simulink model "svpwm"  (R2022b)
settings: Solver=FixedStepAuto  StartTime=0.0  StopTime=10.0  FixedStep=1e-4  RelTol=1e-3
undefined symbols (not defined in the file): Pn
libraries: mcbplantlib x1, autolibpmsmexterior x1
settings Model: DataDictionary=svpwm.sldd  Creator=SSC  LastModifiedBy=SSC
settings OptimizationCC: DefaultParameterBehavior=Inlined  UseDivisionForNetSlopeComputation=on  GainParamInheritBuiltInType=on  UseFloatMulNetSlope=on  InlineInvariantSignals=on  PassReuseOutputArgsAs=Individual arguments  ZeroExternalMemoryAtStartup=off  ZeroInternalMemoryAtStartup=off  NoFixptDivByZeroProtection=on  EfficientFloat2IntCast=on  LifeSpan=1  OptimizeBlockOrder=speed  DifferentSizesBufferReuse=on  EfficientTunableParamExpr=on
settings DebuggingCC: ParameterTunabilityLossMsg=error
settings HardwareCC: ProdBitPerPointer=32  ProdBitPerSizeT=32  ProdBitPerPtrDiffT=32  ProdLargestAtomicInteger=Long  ProdLargestAtomicFloat=Double  ProdWordSize=32  ProdLongLongMode=on  ProdHWDeviceType=ARM Compatible->ARM Cortex-M
settings SFSimCC: MATLABDynamicMemAlloc=off
settings RTWCC: Description=Embedded Coder  SystemTargetFile=ert.tlc  TemplateMakefile=ert_default_tmf  GenerateReport=on  LaunchReport=on
settings CodeAppCC: ForceParamTrailComments=on  IgnoreCustomStorageClasses=off  OperatorAnnotations=on  SimulinkDataObjDesc=on  SFDataObjDesc=on  CustomSymbolStrGlobalVar=rt$N$M  CustomSymbolStrType=$N$M  CustomSymbolStrFcn=$N$M$F  CustomSymbolStrMacro=$N$M  InsertBlockDesc=on
settings ERTTargetCC: TargetLangStandard=C99 (ISO)  CodeReplacementLibrary=ARM Cortex-M  GenerateSampleERTMain=on  IncludeMdlTerminateFcn=off  CombineSignalStateStructs=on  SuppressErrorStatus=on  SupportAbsoluteTime=off  SupportNonFinite=off  SupportComplex=off  InlinedParameterPlacement=NonHierarchical  ERTCustomFileTemplate=example_file_process.tlc  ERTFilePackagingFormat=CompactWithDataFile

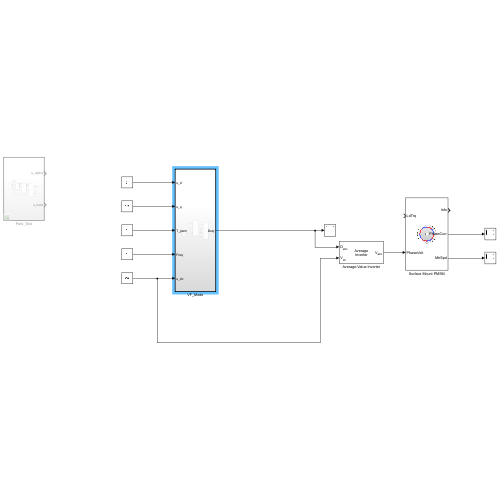
[thumbnail: Simulink's stored preview of the top-level diagram]
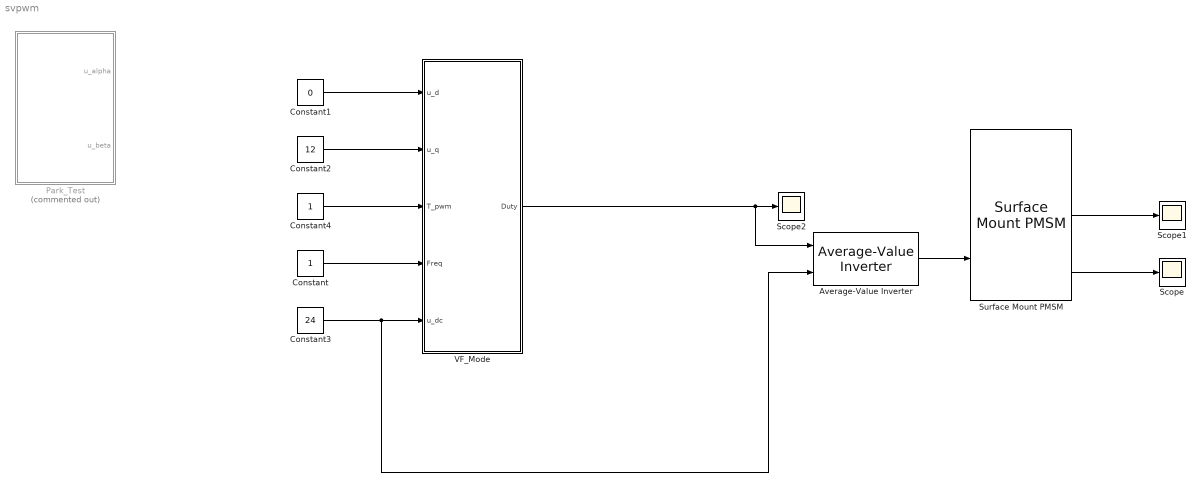
== system svpwm ==
  Average-Value Inverter : mcbplantlib/Average-Value Inverter
      settings: LibrarySourceBlock=mcblib/Electrical Systems/Inverters/Average-Value Inverter
  Constant : Constant
  Constant1 : Constant  Value=0
  Constant2 : Constant  Value=12
  Constant3 : Constant  Value=24
  Constant4 : Constant
  Park_Test : Subsystem  Commented=on  TreatAsAtomicUnit=on
  Scope : Scope
  Scope1 : Scope
  Scope2 : Scope
  Surface Mount PMSM : autolibpmsmexterior/Surface Mount PMSM  port_config=Torque  sim_type=Discrete  Ts=1e-4  P=Pn  Rs=Rs  Ldq_=L  KConstText=Permanent flux linkage constant (lambda_pm):  lambda_pm=flux  Ke=223  Kt=1.323  mechanical=[75e-6,8e-5,0]  idq0=[0 0]  theta_init=0  omega_init=0  KConst=flux  lambda_pm_calc=flux  RefBlkName='autolibpmsmexterior/Surface Mount PMSM'  aMode=5  Ldq="[0.0017      0.0017]"
  VF_Mode : Subsystem  TreatAsAtomicUnit=on
  wires:
  Constant3/1 -> Average-Value Inverter/2, VF_Mode/5(u_dc)
  Average-Value Inverter/1 -> Surface Mount PMSM/2
  Surface Mount PMSM/3 -> Scope/1
  Surface Mount PMSM/2 -> Scope1/1
  VF_Mode/1(Duty) -> Average-Value Inverter/1, Scope2/1
  Constant1/1 -> VF_Mode/1(u_d)
  Constant2/1 -> VF_Mode/2(u_q)
  Constant4/1 -> VF_Mode/3(T_pwm)
  Constant/1 -> VF_Mode/4(Freq)

== system svpwm/Park_Test ==
  AntiPark : Subsystem
  Clark : Subsystem
  Park : Subsystem
  Scope : Scope  NumInputPorts=3
  Scope1 : Scope  NumInputPorts=2
  Scope2 : Scope  NumInputPorts=2
  Scope3 : Scope  NumInputPorts=2
  ThreePhaseCurrGenerator : Subsystem
  u_alpha : Outport
  u_beta : Outport  Port=2
  wires:
  ThreePhaseCurrGenerator/1(ia) -> Scope/1, Clark/1(I_a)  "i_a"
  Clark/2(I_beta) -> Scope1/2, Park/2(i_beta)  "i_beta"
  Clark/1(I_alpha) -> Scope1/1, Park/1(i_alpha)  "i_alpha"
  ThreePhaseCurrGenerator/3(ic) -> Scope/3, Clark/3(I_c)  "i_c"
  ThreePhaseCurrGenerator/2(ib) -> Scope/2, Clark/2(I_b)  "i_b"
  ThreePhaseCurrGenerator/4(electric_theta) -> AntiPark/3(electric_theta), Park/3(electric_theta)  "electric_theta"
  Park/2(i_q) -> Scope3/2, AntiPark/2(u_q)  "i_q"
  Park/1(i_d) -> Scope3/1, AntiPark/1(u_d)  "i_d"
  AntiPark/1(u_alpha) -> u_alpha/1, Scope2/1
  AntiPark/2(u_beta) -> u_beta/1, Scope2/2

== system svpwm/VF_Mode ==
  u_d : Inport
  u_q : Inport  Port=2
  T_pwm : Inport  Port=3
  Freq : Inport  Port=4
  u_dc : Inport  Port=5
  AntiPark : Subsystem
  SVPWM : Subsystem
  ThreePhaseCurrGenerator : Subsystem
  Duty : Outport
  wires:
  u_dc/1 -> SVPWM/4(u_dc)
  ThreePhaseCurrGenerator/1(electric_theta) -> AntiPark/3(electric_theta)  "electric_theta"
  T_pwm/1 -> SVPWM/3(T_pwm)
  SVPWM/1(Duty) -> Duty/1
  u_q/1 -> AntiPark/2(u_q)
  AntiPark/2(u_beta) -> SVPWM/2(U_beta)
  Freq/1 -> ThreePhaseCurrGenerator/1(Freq)
  u_d/1 -> AntiPark/1(u_d)
  AntiPark/1(u_alpha) -> SVPWM/1(U_alpha)

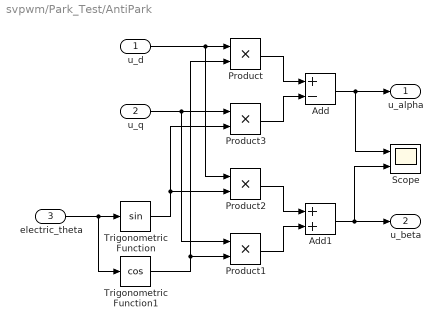
== system svpwm/Park_Test/AntiPark ==
  u_d : Inport
  u_q : Inport  Port=2
  electric_theta : Inport  Port=3
  Add : Sum  Inputs=+-
  Add1 : Sum
  Product{,1..3} (4 alike) : Product
  Scope : Scope  NumInputPorts=2
  Trigonometric Function : Trigonometry
  Trigonometric Function1 : Trigonometry  Operator=cos
  u_alpha : Outport
  u_beta : Outport  Port=2
  wires:
  electric_theta/1 -> Trigonometric Function1/1, Trigonometric Function/1
  u_d/1 -> Product2/1, Product/1
  Trigonometric Function1/1 -> Product/2, Product1/2
  u_q/1 -> Product1/1, Product3/1
  Trigonometric Function/1 -> Product2/2, Product3/2
  Product/1 -> Add/1
  Product3/1 -> Add/2
  Add/1 -> Scope/1, u_alpha/1
  Product2/1 -> Add1/1
  Product1/1 -> Add1/2
  Add1/1 -> Scope/2, u_beta/1

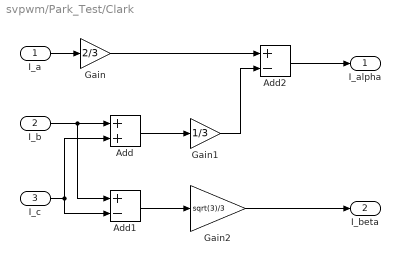
== system svpwm/Park_Test/Clark ==
  I_a : Inport
  I_b : Inport  Port=2
  I_c : Inport  Port=3
  Add : Sum
  Add1 : Sum  Inputs=+-
  Add2 : Sum  Inputs=+-
  Gain : Gain  Gain=2/3
  Gain1 : Gain  Gain=1/3
  Gain2 : Gain  Gain=sqrt(3)/3
  I_alpha : Outport
  I_beta : Outport  Port=2
  wires:
  I_a/1 -> Gain/1
  I_b/1 -> Add1/1, Add/1
  I_c/1 -> Add/2, Add1/2
  Add/1 -> Gain1/1
  Add1/1 -> Gain2/1
  Gain/1 -> Add2/1
  Gain1/1 -> Add2/2
  Add2/1 -> I_alpha/1
  Gain2/1 -> I_beta/1

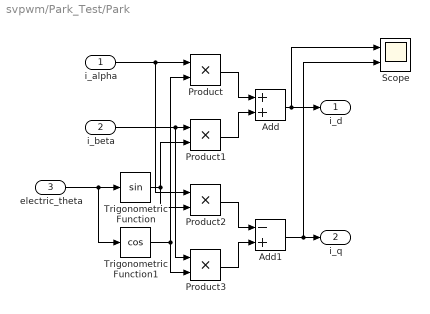
== system svpwm/Park_Test/Park ==
  i_alpha : Inport
  i_beta : Inport  Port=2
  electric_theta : Inport  Port=3
  Add : Sum
  Add1 : Sum  Inputs=-+
  Product{,1..3} (4 alike) : Product
  Scope : Scope  NumInputPorts=2
  Trigonometric Function : Trigonometry
  Trigonometric Function1 : Trigonometry  Operator=cos
  i_d : Outport
  i_q : Outport  Port=2
  wires:
  electric_theta/1 -> Trigonometric Function1/1, Trigonometric Function/1
  i_alpha/1 -> Product2/1, Product/1
  Trigonometric Function1/1 -> Product3/2, Product/2
  i_beta/1 -> Product3/1, Product1/1
  Trigonometric Function/1 -> Product2/2, Product1/2
  Product/1 -> Add/1
  Product1/1 -> Add/2
  Product2/1 -> Add1/1
  Product3/1 -> Add1/2
  Add/1 -> Scope/1, i_d/1
  Add1/1 -> Scope/2, i_q/1

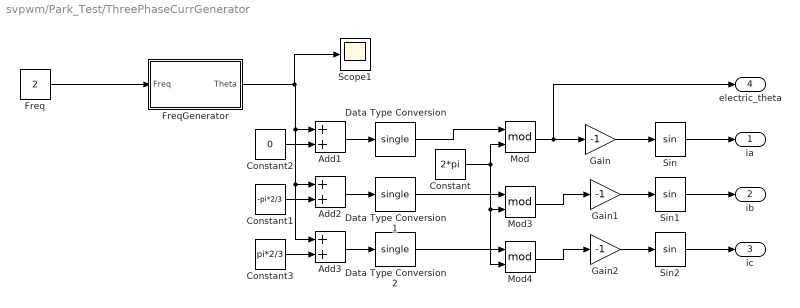
== system svpwm/Park_Test/ThreePhaseCurrGenerator ==
  Add1 : Sum  AccumDataTypeStr=single  OutDataTypeStr=single
  Add2 : Sum  AccumDataTypeStr=single  OutDataTypeStr=single
  Add3 : Sum  AccumDataTypeStr=single  OutDataTypeStr=single
  Constant : Constant  Value=2*pi  OutDataTypeStr=single
  Constant1 : Constant  Value=-pi*2/3  OutDataTypeStr=single
  Constant2 : Constant  Value=0  OutDataTypeStr=single
  Constant3 : Constant  Value=pi*2/3  OutDataTypeStr=single
  Data Type Conversion : DataTypeConversion  OutDataTypeStr=single  SaturateOnIntegerOverflow=off  RndMeth=Floor
  Data Type Conversion1 : DataTypeConversion  OutDataTypeStr=single  SaturateOnIntegerOverflow=off  RndMeth=Floor
  Data Type Conversion2 : DataTypeConversion  OutDataTypeStr=single  SaturateOnIntegerOverflow=off  RndMeth=Floor
  Freq : Constant  Value=2  OutDataTypeStr=single
  FreqGenerator : Subsystem
  Gain : Gain  Gain=-1
  Gain1 : Gain  Gain=-1
  Gain2 : Gain  Gain=-1
  Mod : Math  Operator=mod
  Mod3 : Math  Operator=mod
  Mod4 : Math  Operator=mod
  Scope1 : Scope
  Sin : Trigonometry  ApproximationMethod=Lookup
  Sin1 : Trigonometry  ApproximationMethod=Lookup
  Sin2 : Trigonometry  ApproximationMethod=Lookup
  ia : Outport
  ib : Outport  Port=2
  ic : Outport  Port=3
  electric_theta : Outport  Port=4
  wires:
  Sin2/1 -> ic/1
  Constant2/1 -> Add1/2
  Mod/1 -> electric_theta/1, Gain/1
  Constant/1 -> Mod4/2, Mod3/2, Mod/2
  Constant3/1 -> Add3/2
  Gain2/1 -> Sin2/1
  Constant1/1 -> Add2/2
  FreqGenerator/1(Theta) -> Scope1/1, Add3/1, Add2/1, Add1/1
  Sin/1 -> ia/1
  Sin1/1 -> ib/1
  Gain/1 -> Sin/1
  Add1/1 -> Data Type Conversion/1
  Data Type Conversion1/1 -> Mod3/1
  Mod3/1 -> Gain1/1
  Data Type Conversion/1 -> Mod/1
  Add2/1 -> Data Type Conversion1/1
  Add3/1 -> Data Type Conversion2/1
  Freq/1 -> FreqGenerator/1(Freq)
  Gain1/1 -> Sin1/1
  Data Type Conversion2/1 -> Mod4/1
  Mod4/1 -> Gain2/1

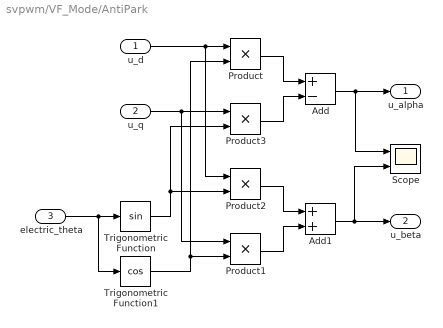
== system svpwm/VF_Mode/AntiPark ==
  u_d : Inport
  u_q : Inport  Port=2
  electric_theta : Inport  Port=3
  Add : Sum  Inputs=+-
  Add1 : Sum
  Product{,1..3} (4 alike) : Product
  Scope : Scope  NumInputPorts=2
  Trigonometric Function : Trigonometry
  Trigonometric Function1 : Trigonometry  Operator=cos
  u_alpha : Outport
  u_beta : Outport  Port=2
  wires:
  electric_theta/1 -> Trigonometric Function1/1, Trigonometric Function/1
  u_d/1 -> Product2/1, Product/1
  Trigonometric Function1/1 -> Product/2, Product1/2
  u_q/1 -> Product1/1, Product3/1
  Trigonometric Function/1 -> Product2/2, Product3/2
  Product/1 -> Add/1
  Product3/1 -> Add/2
  Add/1 -> Scope/1, u_alpha/1
  Product2/1 -> Add1/1
  Product1/1 -> Add1/2
  Add1/1 -> Scope/2, u_beta/1

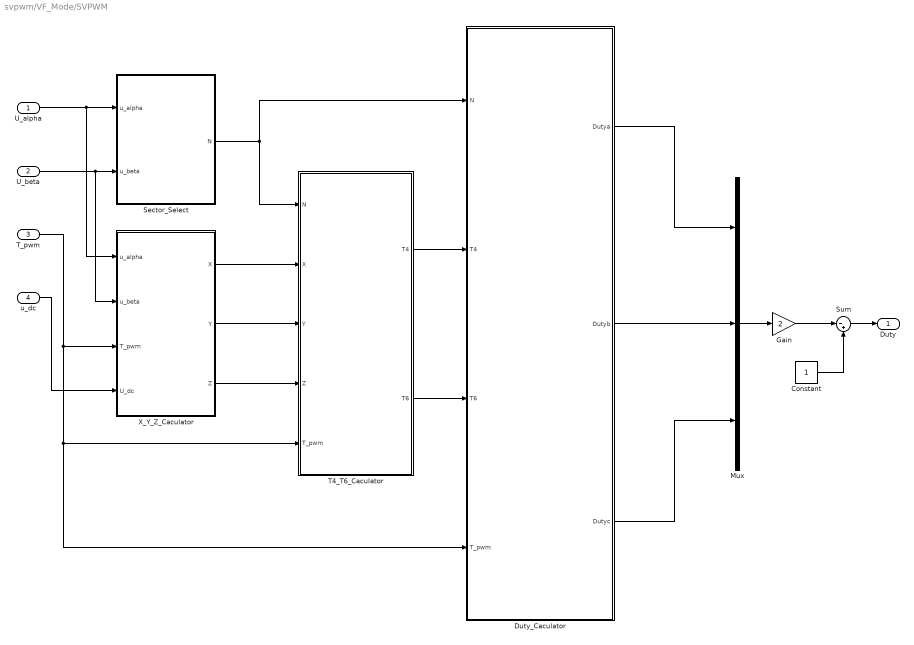
== system svpwm/VF_Mode/SVPWM ==
  U_alpha : Inport
  U_beta : Inport  Port=2
  T_pwm : Inport  Port=3
  u_dc : Inport  Port=4
  Constant : Constant
  Duty_Caculator : Subsystem
  Gain : Gain  Gain=2
  Mux : Mux  Inputs=3
  Sector_Select : Subsystem
  Sum : Sum  Inputs=|-+
  T4_T6_Caculator : Subsystem
  X_Y_Z_Caculator : Subsystem
  Duty : Outport
  wires:
  U_alpha/1 -> X_Y_Z_Caculator/1(u_alpha), Sector_Select/1(u_alpha)
  U_beta/1 -> X_Y_Z_Caculator/2(u_beta), Sector_Select/2(u_beta)
  T_pwm/1 -> Duty_Caculator/4(T_pwm), T4_T6_Caculator/5(T_pwm), X_Y_Z_Caculator/3(T_pwm)
  u_dc/1 -> X_Y_Z_Caculator/4(U_dc)
  X_Y_Z_Caculator/1(X) -> T4_T6_Caculator/2(X)
  X_Y_Z_Caculator/2(Y) -> T4_T6_Caculator/3(Y)
  X_Y_Z_Caculator/3(Z) -> T4_T6_Caculator/4(Z)
  Sector_Select/1(N) -> T4_T6_Caculator/1(N), Duty_Caculator/1(N)
  T4_T6_Caculator/2(T6) -> Duty_Caculator/3(T6)
  T4_T6_Caculator/1(T4) -> Duty_Caculator/2(T4)
  Duty_Caculator/2(Dutyb) -> Mux/2
  Duty_Caculator/1(Dutya) -> Mux/1
  Duty_Caculator/3(Dutyc) -> Mux/3
  Sum/1 -> Duty/1
  Constant/1 -> Sum/2
  Mux/1 -> Gain/1
  Gain/1 -> Sum/1

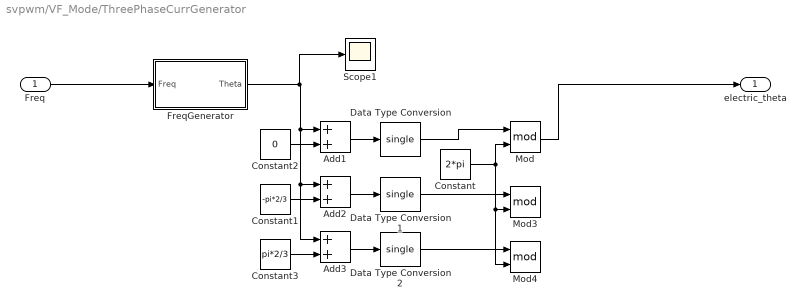
== system svpwm/VF_Mode/ThreePhaseCurrGenerator ==
  Freq : Inport
  Add1 : Sum  AccumDataTypeStr=single  OutDataTypeStr=single
  Add2 : Sum  AccumDataTypeStr=single  OutDataTypeStr=single
  Add3 : Sum  AccumDataTypeStr=single  OutDataTypeStr=single
  Constant : Constant  Value=2*pi  OutDataTypeStr=single
  Constant1 : Constant  Value=-pi*2/3  OutDataTypeStr=single
  Constant2 : Constant  Value=0  OutDataTypeStr=single
  Constant3 : Constant  Value=pi*2/3  OutDataTypeStr=single
  Data Type Conversion : DataTypeConversion  OutDataTypeStr=single  SaturateOnIntegerOverflow=off  RndMeth=Floor
  Data Type Conversion1 : DataTypeConversion  OutDataTypeStr=single  SaturateOnIntegerOverflow=off  RndMeth=Floor
  Data Type Conversion2 : DataTypeConversion  OutDataTypeStr=single  SaturateOnIntegerOverflow=off  RndMeth=Floor
  FreqGenerator : Subsystem
  Mod : Math  Operator=mod
  Mod3 : Math  Operator=mod
  Mod4 : Math  Operator=mod
  Scope1 : Scope
  electric_theta : Outport
  wires:
  Constant2/1 -> Add1/2
  Mod/1 -> electric_theta/1
  Constant/1 -> Mod4/2, Mod3/2, Mod/2
  Constant3/1 -> Add3/2
  Constant1/1 -> Add2/2
  FreqGenerator/1(Theta) -> Scope1/1, Add3/1, Add2/1, Add1/1
  Add1/1 -> Data Type Conversion/1
  Data Type Conversion1/1 -> Mod3/1
  Data Type Conversion/1 -> Mod/1
  Add2/1 -> Data Type Conversion1/1
  Add3/1 -> Data Type Conversion2/1
  Freq/1 -> FreqGenerator/1(Freq)
  Data Type Conversion2/1 -> Mod4/1

== system svpwm/Park_Test/ThreePhaseCurrGenerator/FreqGenerator ==
  Freq : Inport
  Gain : Gain  Gain=1/10e3*2*pi  OutDataTypeStr=single
  RangeLimit : Subsystem
  Sum : Sum  Inputs=|++  OutDataTypeStr=Inherit: Same as first input
  Unit Delay : UnitDelay  SampleTime=-1  HasFrameUpgradeWarning=on
  Theta : Outport
  wires:
  Freq/1 -> Gain/1
  RangeLimit/1(Theta) -> Theta/1, Unit Delay/1
  Gain/1 -> Sum/1
  Sum/1 -> RangeLimit/1(In)
  Unit Delay/1 -> Sum/2

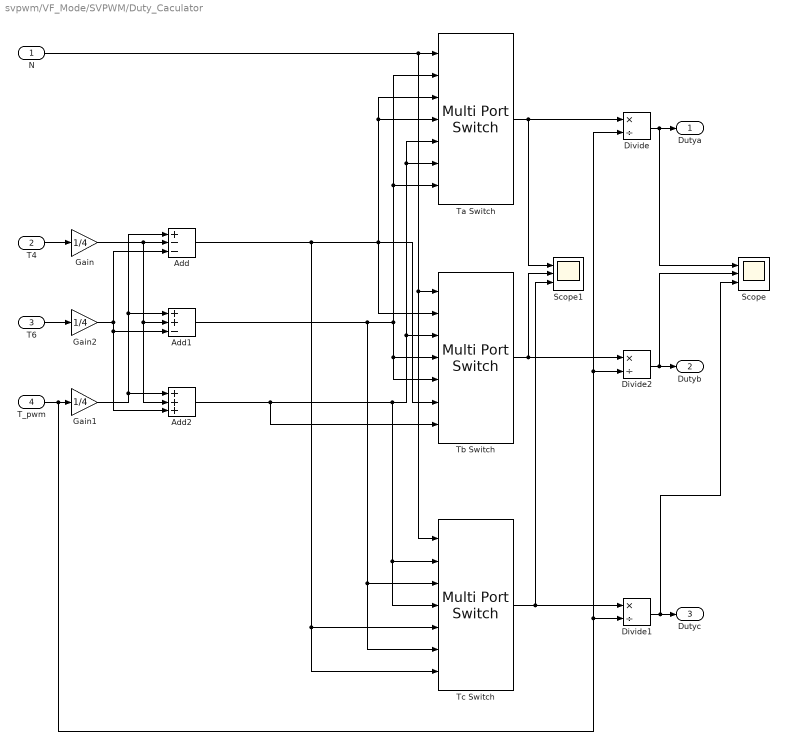
== system svpwm/VF_Mode/SVPWM/Duty_Caculator ==
  N : Inport
  T4 : Inport  Port=2
  T6 : Inport  Port=3
  T_pwm : Inport  Port=4
  Add : Sum  Inputs=+--
  Add1 : Sum  Inputs=++-
  Add2 : Sum  Inputs=+++
  Divide : Product  Inputs=*/
  Divide1 : Product  Inputs=*/
  Divide2 : Product  Inputs=*/
  Gain : Gain  Gain=1/4
  Gain1 : Gain  Gain=1/4
  Gain2 : Gain  Gain=1/4
  Scope : Scope  NumInputPorts=3
  Scope1 : Scope  NumInputPorts=3
  Ta Switch : MultiPortSwitch  Inputs=6  SaturateOnIntegerOverflow=off  InputSameDT=off
  Tb Switch : MultiPortSwitch  Inputs=6  SaturateOnIntegerOverflow=off  InputSameDT=off
  Tc Switch : MultiPortSwitch  Inputs=6  SaturateOnIntegerOverflow=off  InputSameDT=off
  Dutya : Outport
  Dutyb : Outport  Port=2
  Dutyc : Outport  Port=3
  wires:
  T4/1 -> Gain/1
  T6/1 -> Gain2/1
  T_pwm/1 -> Divide2/2, Divide/2, Divide1/2, Gain1/1
  Gain1/1 -> Add2/1, Add1/1, Add/1
  Gain/1 -> Add2/2, Add1/2, Add/2
  Gain2/1 -> Add2/3, Add1/3, Add/3
  N/1 -> Tc Switch/1, Tb Switch/1, Ta Switch/1
  Add/1 -> Tc Switch/7, Tc Switch/5, Tb Switch/6, Ta Switch/3, Ta Switch/4, Tb Switch/2
  Add1/1 -> Tc Switch/3, Tc Switch/6, Ta Switch/7, Ta Switch/2, Tb Switch/5, Tb Switch/4
  Add2/1 -> Tb Switch/7, Ta Switch/5, Ta Switch/6, Tb Switch/3, Tc Switch/4, Tc Switch/2
  Ta Switch/1 -> Scope1/1, Divide/1
  Tb Switch/1 -> Scope1/2, Divide2/1
  Tc Switch/1 -> Scope1/3, Divide1/1
  Divide/1 -> Scope/1, Dutya/1
  Divide1/1 -> Scope/3, Dutyc/1
  Divide2/1 -> Scope/2, Dutyb/1

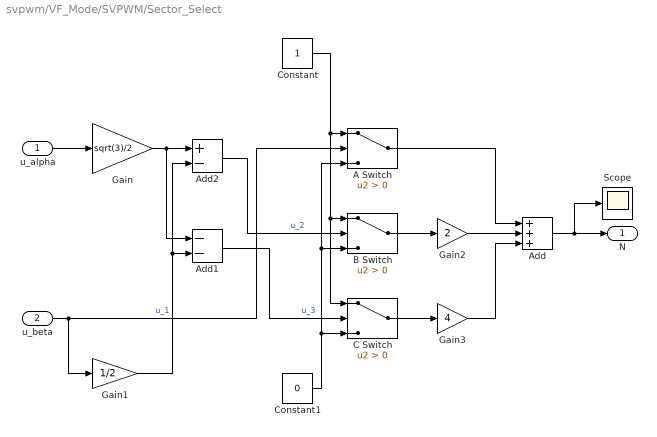
== system svpwm/VF_Mode/SVPWM/Sector_Select ==
  u_alpha : Inport
  u_beta : Inport  Port=2
  " A Switch" : Switch  Criteria=u2 > Threshold  SaturateOnIntegerOverflow=off  InputSameDT=off
  " B Switch" : Switch  Criteria=u2 > Threshold  SaturateOnIntegerOverflow=off  InputSameDT=off
  " C Switch" : Switch  Criteria=u2 > Threshold  SaturateOnIntegerOverflow=off  InputSameDT=off
  Add : Sum  Inputs=+++
  Add1 : Sum  Inputs=--
  Add2 : Sum  Inputs=+-
  Constant : Constant
  Constant1 : Constant  Value=0
  Gain : Gain  Gain=sqrt(3)/2
  Gain1 : Gain  Gain=1/2
  Gain2 : Gain  Gain=2
  Gain3 : Gain  Gain=4
  Scope : Scope
  N : Outport
  wires:
  Constant/1 -> " C Switch"/1, " B Switch"/1, " A Switch"/1
  Constant1/1 -> " C Switch"/3, " B Switch"/3, " A Switch"/3
  " A Switch"/1 -> Add/1
  Add/1 -> Scope/1, N/1
  " C Switch"/1 -> Gain3/1
  " B Switch"/1 -> Gain2/1
  u_beta/1 -> Gain1/1, " A Switch"/2  "u_1"
  u_alpha/1 -> Gain/1
  Gain/1 -> Add1/1, Add2/1
  Gain1/1 -> Add1/2, Add2/2
  Add2/1 -> " B Switch"/2  "u_2"
  Add1/1 -> " C Switch"/2  "u_3"
  Gain2/1 -> Add/2
  Gain3/1 -> Add/3

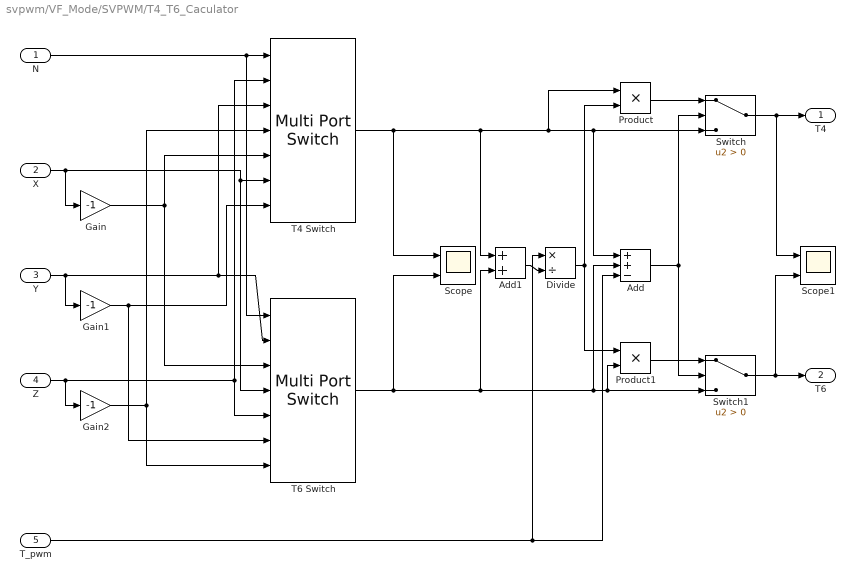
== system svpwm/VF_Mode/SVPWM/T4_T6_Caculator ==
  N : Inport
  X : Inport  Port=2
  Y : Inport  Port=3
  Z : Inport  Port=4
  T_pwm : Inport  Port=5
  Add : Sum  Inputs=++-
  Add1 : Sum
  Divide : Product  Inputs=*/
  Gain : Gain  Gain=-1
  Gain1 : Gain  Gain=-1
  Gain2 : Gain  Gain=-1
  Product : Product
  Product1 : Product
  Scope : Scope  NumInputPorts=2
  Scope1 : Scope  NumInputPorts=2
  Switch : Switch  Criteria=u2 > Threshold  SaturateOnIntegerOverflow=off  InputSameDT=off
  Switch1 : Switch  Criteria=u2 > Threshold  SaturateOnIntegerOverflow=off  InputSameDT=off
  T4 Switch : MultiPortSwitch  Inputs=6  SaturateOnIntegerOverflow=off  InputSameDT=off
  T6 Switch : MultiPortSwitch  Inputs=6  SaturateOnIntegerOverflow=off  InputSameDT=off
  T4 : Outport
  T6 : Outport  Port=2
  wires:
  Z/1 -> T4 Switch/2, T6 Switch/5, Gain2/1
  Y/1 -> Gain1/1, T4 Switch/3, T6 Switch/2
  X/1 -> T4 Switch/6, T6 Switch/4, Gain/1
  N/1 -> T6 Switch/1, T4 Switch/1
  Gain/1 -> T6 Switch/3, T4 Switch/5
  Gain2/1 -> T6 Switch/7, T4 Switch/4
  Gain1/1 -> T4 Switch/7, T6 Switch/6
  T4 Switch/1 -> Add1/1, Product/1, Add/1, Switch/3, Scope/1
  T6 Switch/1 -> Add1/2, Add/2, Switch1/3, Product1/2, Scope/2
  T_pwm/1 -> Add/3, Divide/1
  Add/1 -> Switch1/2, Switch/2
  Add1/1 -> Divide/2
  Product1/1 -> Switch1/1
  Product/1 -> Switch/1
  Divide/1 -> Product/2, Product1/1
  Switch/1 -> Scope1/1, T4/1
  Switch1/1 -> Scope1/2, T6/1

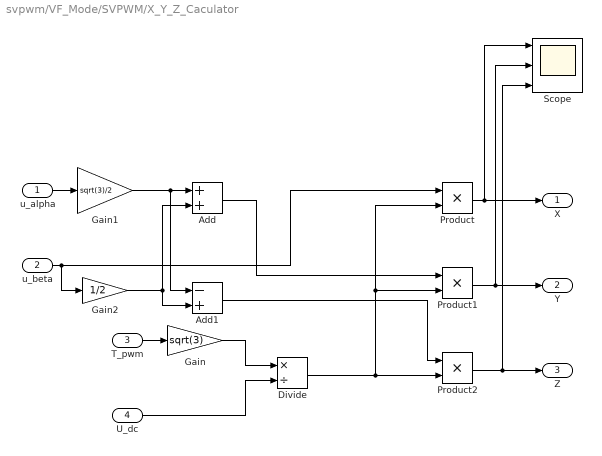
== system svpwm/VF_Mode/SVPWM/X_Y_Z_Caculator ==
  u_alpha : Inport
  u_beta : Inport  Port=2
  T_pwm : Inport  Port=3
  U_dc : Inport  Port=4
  Add : Sum
  Add1 : Sum  Inputs=-+
  Divide : Product  Inputs=*/
  Gain : Gain  Gain=sqrt(3)
  Gain1 : Gain  Gain=sqrt(3)/2
  Gain2 : Gain  Gain=1/2
  Product : Product
  Product1 : Product
  Product2 : Product
  Scope : Scope  NumInputPorts=3
  X : Outport
  Y : Outport  Port=2
  Z : Outport  Port=3
  wires:
  T_pwm/1 -> Gain/1
  U_dc/1 -> Divide/2
  Gain/1 -> Divide/1
  u_beta/1 -> Gain2/1, Product/1
  Divide/1 -> Product2/2, Product1/2, Product/2
  Product/1 -> Scope/1, X/1
  u_alpha/1 -> Gain1/1
  Gain1/1 -> Add1/1, Add/1
  Gain2/1 -> Add1/2, Add/2
  Add/1 -> Product1/1
  Product1/1 -> Scope/2, Y/1
  Add1/1 -> Product2/1
  Product2/1 -> Scope/3, Z/1

== system svpwm/VF_Mode/ThreePhaseCurrGenerator/FreqGenerator ==
  Freq : Inport
  Gain : Gain  Gain=1/10e3*2*pi  OutDataTypeStr=single
  RangeLimit : Subsystem
  Sum : Sum  Inputs=|++  OutDataTypeStr=Inherit: Same as first input
  Unit Delay : UnitDelay  SampleTime=-1  HasFrameUpgradeWarning=on
  Theta : Outport
  wires:
  Freq/1 -> Gain/1
  RangeLimit/1(Theta) -> Theta/1, Unit Delay/1
  Gain/1 -> Sum/1
  Sum/1 -> RangeLimit/1(In)
  Unit Delay/1 -> Sum/2

== system svpwm/Park_Test/ThreePhaseCurrGenerator/FreqGenerator/RangeLimit ==
  In : Inport
  Constant : Constant  Value=2*pi  OutDataTypeStr=single  SampleTime=-1
  Constant1 : Constant  Value=0  OutDataTypeStr=single  SampleTime=-1
  If : If  NumInputs=2  IfExpression=u1  ElseIfExpressions=u2
  If Action Subsystem1 : Subsystem  TreatAsAtomicUnit=on
  If Action Subsystem2 : Subsystem  TreatAsAtomicUnit=on
  If Action Subsystem3 : Subsystem  TreatAsAtomicUnit=on
  Merge : Merge  Inputs=3
  Relational Operator : RelationalOperator  Operator=>  OutDataTypeStr=boolean  RndMeth=Simplest  InputSameDT=off
  Relational Operator1 : RelationalOperator  Operator=<  OutDataTypeStr=boolean  RndMeth=Simplest  InputSameDT=off
  Theta : Outport
  wires:
  Relational Operator/1 -> If/1
  Constant/1 -> Relational Operator/2
  In/1 -> Relational Operator1/1, If Action Subsystem2/1(In1), If Action Subsystem3/1(In1), If Action Subsystem1/1(In1), Relational Operator/1
  Merge/1 -> Theta/1
  If/3 -> If Action Subsystem2/Action
  If/1 -> If Action Subsystem1/Action
  If Action Subsystem2/1(Out1) -> Merge/1
  Constant1/1 -> Relational Operator1/2
  Relational Operator1/1 -> If/2
  If/2 -> If Action Subsystem3/Action
  If Action Subsystem1/1(Out1) -> Merge/3
  If Action Subsystem3/1(Out1) -> Merge/2

== system svpwm/VF_Mode/ThreePhaseCurrGenerator/FreqGenerator/RangeLimit ==
  In : Inport
  Constant : Constant  Value=2*pi  OutDataTypeStr=single  SampleTime=-1
  Constant1 : Constant  Value=0  OutDataTypeStr=single  SampleTime=-1
  If : If  NumInputs=2  IfExpression=u1  ElseIfExpressions=u2
  If Action Subsystem1 : Subsystem  TreatAsAtomicUnit=on
  If Action Subsystem2 : Subsystem  TreatAsAtomicUnit=on
  If Action Subsystem3 : Subsystem  TreatAsAtomicUnit=on
  Merge : Merge  Inputs=3
  Relational Operator : RelationalOperator  Operator=>  OutDataTypeStr=boolean  RndMeth=Simplest  InputSameDT=off
  Relational Operator1 : RelationalOperator  Operator=<  OutDataTypeStr=boolean  RndMeth=Simplest  InputSameDT=off
  Theta : Outport
  wires:
  Relational Operator/1 -> If/1
  Constant/1 -> Relational Operator/2
  In/1 -> Relational Operator1/1, If Action Subsystem2/1(In1), If Action Subsystem3/1(In1), If Action Subsystem1/1(In1), Relational Operator/1
  Merge/1 -> Theta/1
  If/3 -> If Action Subsystem2/Action
  If/1 -> If Action Subsystem1/Action
  If Action Subsystem2/1(Out1) -> Merge/1
  Constant1/1 -> Relational Operator1/2
  Relational Operator1/1 -> If/2
  If/2 -> If Action Subsystem3/Action
  If Action Subsystem1/1(Out1) -> Merge/3
  If Action Subsystem3/1(Out1) -> Merge/2

== system svpwm/Park_Test/ThreePhaseCurrGenerator/FreqGenerator/RangeLimit/If Action Subsystem1 ==
  In1 : Inport
  Action Port : ActionPort  ActionPortLabel=if(u1)
  Constant : Constant  Value=2*pi  OutDataTypeStr=single  SampleTime=-1
  Sum : Sum  Inputs=|+-
  Out1 : Outport
  wires:
  In1/1 -> Sum/1
  Constant/1 -> Sum/2
  Sum/1 -> Out1/1

== system svpwm/Park_Test/ThreePhaseCurrGenerator/FreqGenerator/RangeLimit/If Action Subsystem2 ==
  In1 : Inport
  Action Port : ActionPort  ActionPortLabel=else
  Out1 : Outport
  wires:
  In1/1 -> Out1/1

== system svpwm/Park_Test/ThreePhaseCurrGenerator/FreqGenerator/RangeLimit/If Action Subsystem3 ==
  In1 : Inport
  Action Port : ActionPort  ActionPortLabel=elseif(u2)
  Constant : Constant  Value=2*pi  OutDataTypeStr=single  SampleTime=-1
  Sum : Sum  Inputs=|++
  Out1 : Outport
  wires:
  Constant/1 -> Sum/2
  In1/1 -> Sum/1
  Sum/1 -> Out1/1

== system svpwm/VF_Mode/ThreePhaseCurrGenerator/FreqGenerator/RangeLimit/If Action Subsystem1 ==
  In1 : Inport
  Action Port : ActionPort  ActionPortLabel=if(u1)
  Constant : Constant  Value=2*pi  OutDataTypeStr=single  SampleTime=-1
  Sum : Sum  Inputs=|+-
  Out1 : Outport
  wires:
  In1/1 -> Sum/1
  Constant/1 -> Sum/2
  Sum/1 -> Out1/1

== system svpwm/VF_Mode/ThreePhaseCurrGenerator/FreqGenerator/RangeLimit/If Action Subsystem2 ==
  In1 : Inport
  Action Port : ActionPort  ActionPortLabel=else
  Out1 : Outport
  wires:
  In1/1 -> Out1/1

== system svpwm/VF_Mode/ThreePhaseCurrGenerator/FreqGenerator/RangeLimit/If Action Subsystem3 ==
  In1 : Inport
  Action Port : ActionPort  ActionPortLabel=elseif(u2)
  Constant : Constant  Value=2*pi  OutDataTypeStr=single  SampleTime=-1
  Sum : Sum  Inputs=|++
  Out1 : Outport
  wires:
  Constant/1 -> Sum/2
  In1/1 -> Sum/1
  Sum/1 -> Out1/1
